simulink model "test"  (R2016a)
settings: Solver=VariableStepAuto  StartTime=0.0  StopTime=10.0  RelTol=1e-3
libraries: vrlib x2
settings Model: Creator=Prajesh Sanghvi  LastModifiedBy=Prajesh Sanghvi

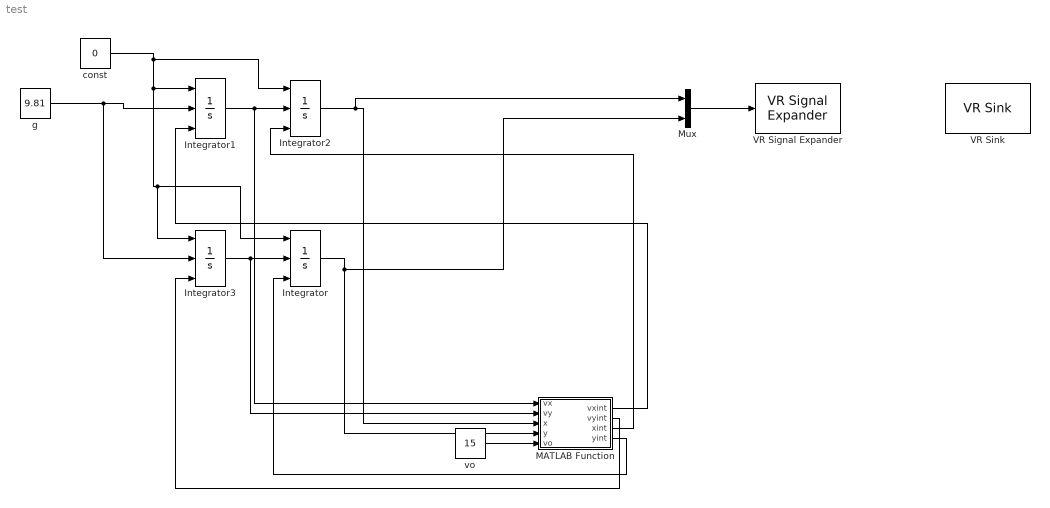
== system test ==
  Integrator{,1..3} (4 alike) : Integrator  ExternalReset=rising  InitialConditionSource=external
  MATLAB Function : MATLAB Function  TreatAsAtomicUnit=on
  Mux : Mux  Inputs=2
  VR Signal Expander : vrlib/VR Signal Expander  outwidth=3  outidx=[1 2]
  VR Sink : vrlib/VR Sink  InstantiateOnLoad=on  SampleTime=0.1  ViewEnable=on  RemoteChange=off  RemoteView=on  AutoView=off  VideoDimensions=[]  AllowVariableSize=off
  const : Constant  Value=0
  g : Constant  Value=9.81
  vo : Constant  Value=15
  wires:
  MATLAB Function/1(vxint) -> Integrator1/3
  MATLAB Function/2(vyint) -> Integrator3/3
  MATLAB Function/3(xint) -> Integrator2/3
  MATLAB Function/4(yint) -> Integrator/3
  Integrator2/1 -> Mux/1, MATLAB Function/3(x)
  Integrator/1 -> Mux/2, MATLAB Function/4(y)
  Integrator1/1 -> MATLAB Function/1(vx), Integrator2/2
  Integrator3/1 -> MATLAB Function/2(vy), Integrator/2
  g/1 -> Integrator3/2, Integrator1/2
  const/1 -> Integrator2/1, Integrator3/1, Integrator/1, Integrator1/1
  vo/1 -> MATLAB Function/5(vo)
  Mux/1 -> VR Signal Expander/1

== matlab function test/MATLAB Function ==
  data: vx input; vxint output; vy input; x input; y input; vyint output; xint output; yint output; vo input
function [vxint,vyint,xint,yint] = fcn(vx,vy,x,y,vo)
%#codegen

vxint=vo*sin(pi/3);
vyint=vo*cos(pi/3);
xint=-6;
yint=0.5;
